simulink model "trackwheelmodel"  (R2021a)
settings: Solver=VariableStepAuto  StartTime=0.0  StopTime=10  RelTol=1e-3
values from neighbouring files (symbols this model uses):
  omegal = 50    [solveequilibrium.m]    (also in vsSim.m = omegalgrid(i))
  omegar = -50    [solveequilibrium.m]    (also in vsSim.m = omegargrid(i))
libraries: autolibshared x1, simulink x1

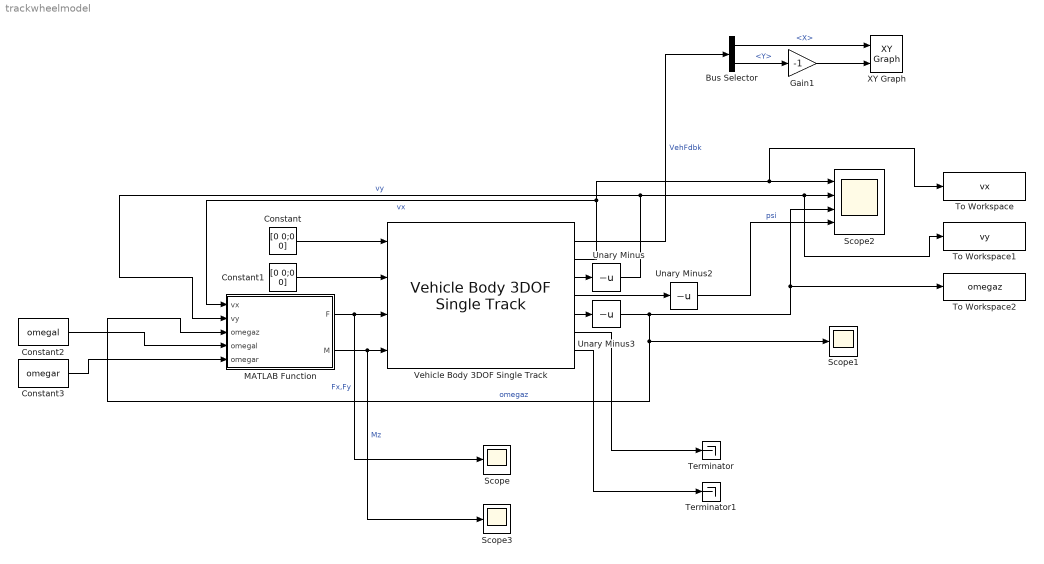
== system trackwheelmodel ==
  Bus Selector : BusSelector  OutputSignals=InertFrm.Cg.Disp.X,InertFrm.Cg.Disp.Y
  Constant : Constant  Value=[0 0;0 0]
  Constant1 : Constant  Value=[0 0;0 0]
  Constant2 : Constant  Value=omegal
  Constant3 : Constant  Value=omegar
  Gain1 : Gain  Gain=-1
  MATLAB Function : MATLAB Function  TreatAsAtomicUnit=on
  Scope : Scope
  Scope1 : Scope
  Scope2 : Scope  NumInputPorts=4
  Scope3 : Scope
  Terminator : Terminator
  Terminator1 : Terminator
  To Workspace : ToWorkspace  VariableName=vx  SaveFormat=Timeseries  SampleTime=-1
  To Workspace1 : ToWorkspace  VariableName=vy  SaveFormat=Timeseries  SampleTime=-1
  To Workspace2 : ToWorkspace  VariableName=omegaz  SaveFormat=Timeseries  SampleTime=-1
  Unary Minus : UnaryMinus
  Unary Minus2 : UnaryMinus
  Unary Minus3 : UnaryMinus
  Vehicle Body 3DOF Single Track : autolibshared/Vehicle Body 3DOF Single Track  trackMode=Dual  inputMode=External forces  frontSteerMode=off  rearSteerMode=off  windMode=off  muMode=off  extFMode=on  extMMode=on  htchFMode=off  htchMMode=off  extXo=off  extpsio=off  extxdoto=off  extro=off  extYo=off  extTamb=off  extydoto=off  aMode=2  NF=2  NR=2  m=2000  a=1.4  b=1.6  h=0.35  dh=1  hh=0.2  X_o=0  xdot_o=5  CalphaMode=off  sigmaMode=on  d=0  hl=0  w=[1.4,1.4]  Cy_f=12e3  Cy_r=11e3  sigma_f=.1  sigma_r=.1  alpha_f_brk=[-.1 .1]  Cy_f_data=[-9e3 9e3]  alpha_r_brk=[-.1 .1]  Cy_r_data=[-9e3 9e3]  Y_o=0  ydot_o=0  Izz=4000  psi_o=0  r_o=0  Af=2  Cd=.3  Cl=.1  Cpm=.1  beta_w=[0:0.01:0.3]  Cs=[0:0.03:0.9]  Cym=[0:0.01:0.3]  Pabs=101325  Tair=273  g=9.81  mu=1  xdot_tol=.01  Fznom=5000  Fxtire_sat=7e4  Fytire_sat=7e4  longOff=0  latOff=0  vertOff=0  wrapAng=off
      settings: SourceProductBaseCode=PW,DR,MT,UV,VE
  XY Graph : simulink/Sinks/XY Graph  xmin=-150  xmax=150  ymin=-200  ymax=100  st=-1
  wires:
  Constant/1 -> Vehicle Body 3DOF Single Track/1
  Constant1/1 -> Vehicle Body 3DOF Single Track/2
  Vehicle Body 3DOF Single Track/2 -> MATLAB Function/1(vx), To Workspace/1, Scope2/1  "vx"
  Constant2/1 -> MATLAB Function/4(omegal)
  Constant3/1 -> MATLAB Function/5(omegar)
  Bus Selector/1 -> XY Graph/1  "<X>"
  Bus Selector/2 -> Gain1/1  "<Y>"
  Vehicle Body 3DOF Single Track/4 -> Unary Minus2/1
  Vehicle Body 3DOF Single Track/5 -> Unary Minus3/1
  Vehicle Body 3DOF Single Track/3 -> Unary Minus/1
  MATLAB Function/2(M) -> Scope3/1, Vehicle Body 3DOF Single Track/4  "Mz"
  MATLAB Function/1(F) -> Scope/1, Vehicle Body 3DOF Single Track/3  "Fx,Fy"
  Vehicle Body 3DOF Single Track/1 -> Bus Selector/1  "VehFdbk"
  Gain1/1 -> XY Graph/2
  Unary Minus3/1 -> MATLAB Function/3(omegaz), Scope1/1, Scope2/3, To Workspace2/1  "omegaz"
  Unary Minus2/1 -> Scope2/4  "psi"
  Unary Minus/1 -> MATLAB Function/2(vy), To Workspace1/1, Scope2/2  "vy"
  Vehicle Body 3DOF Single Track/6 -> Terminator/1
  Vehicle Body 3DOF Single Track/7 -> Terminator1/1

== matlab function trackwheelmodel/MATLAB Function ==
  data: vx input; F output; vy input; omegaz input; omegal input; omegar input; M output
function [F,M] = fcn(vx,vy,omegaz,omegal,omegar)

[Fx,Fy,Mz] = trackforce(vx,vy,omegaz,omegal,omegar);

% MATLAB uses SAE coordinate

F = [Fx -Fy 0];

M = [0 0 -Mz];

end
